simulink model "CrossAR"  (R2020b)
settings: Solver=FixedStepDiscrete  StartTime=0.0  StopTime=99*ModelParam.Samples4Frame  RelTol=1e-3
InitFcn:
  | disp([gcs ': InitFcn']);
  | ModelParam = CrossAR_init([bdroot '/ModelParameters']);
undefined symbols (not defined in the file or in its folder): dfilt
libraries: dspstat3 x17, commchan3 x2, LibCrossAr x2, dspparest3 x2, dspobslib x2, dspsrcs4 x1
Description:
  | % Francesco Conti, Gaetano Scarano, Stefania Colonnese, Mauro Biagi, 2021/01/04%
  | % Copyright: This is published under BSD BSD 3-Clause License
  | 
  | % Copyright (c) 2021, francescoconti748 (Francesco Conti)
  | % All rights reserved, see LICENSE file
  | %
settings Model: Creator=gscarano  LastModifiedBy=conti
settings DataIOCC: LimitDataPoints=on  SaveFormat=Array  SignalLoggingSaveFormat=ModelDataLogs  SaveOutput=off  SignalLogging=off  SaveTime=off  ReturnWorkspaceOutputs=off
settings OptimizationCC: ExpressionDepthLimit=2147483647  LifeSpan=inf
settings DebuggingCC: AlgebraicLoopMsg=error  UnderspecifiedInitializationDetection=Classic  MergeDetectMultiDrivingBlocksExec=none  SolverPrmCheckMsg=warning  SingleTaskRateTransMsg=error  FcnCallInpInsideContextMsg=warning  StateNameClashWarn=warning  SFUnexpectedBacktrackingDiag=warning  SFNoUnconditionalDefaultTransitionDiag=warning  SFExecutionAtInitializationDiag=none  ArithmeticOperatorsInVariantConditions=warning
settings HardwareCC: ProdBitPerPointer=32  ProdBitPerSizeT=32  ProdBitPerPtrDiffT=32  ProdLargestAtomicFloat=None  ProdIntDivRoundTo=Undefined  ProdEndianess=Unspecified  ProdWordSize=32  ProdHWDeviceType=32-bit Generic
settings ModelReferenceCC: PropagateSignalLabelsOutOfModel=off
settings SFSimCC: SimUseLocalCustomCode=off  SimParseCustomCode=off  CustomCodeUndefinedFunction=UseInterfaceOnly
settings RTWCC: RTWUseLocalCustomCode=off
settings CodeAppCC: StateflowObjectComments=on
settings GRTTargetCC: TargetLangStandard=C89/C90 (ANSI)  CombineOutputUpdateFcns=off  GRTInterface=on
settings ConfigComp: CovMetricSettings=dw  CovSaveCumulativeToWorkspaceVar=on  CovSaveSingleToWorkspaceVar=on  CovExternalEMLEnable=off  DVMaxProcessTime=600  DVAutomaticStubbing=off  DVModelCoverageObjectives=MCDC  DVMaxTestCaseSteps=500  DVTestSuiteOptimization=CombinedObjectives  DVDetectActiveLogic=on  DVSaveHarnessModel=on  DVSaveReport=on

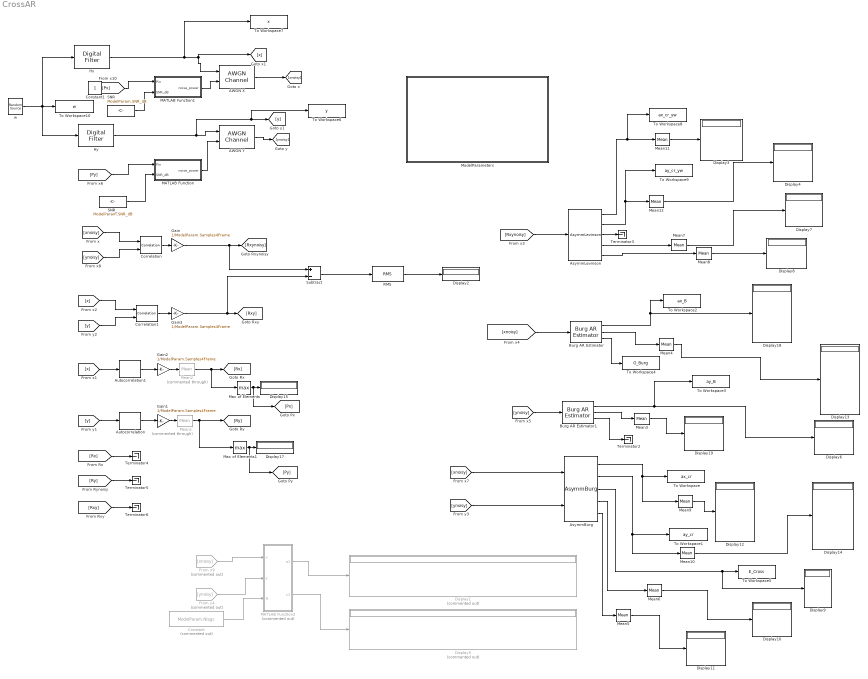
== system CrossAR ==
  AWGN X : commchan3/AWGN Channel  InputProcessing=Columns as channels (frame based)  seed=135  noiseMode=Variance from port  EbNodB=10  EsNodB=10  SNRdB=10  bitsPerSym=1  Ps=1  Tsym=1  variance=ModelParam.NoisePowX
  AWGN Y : commchan3/AWGN Channel  InputProcessing=Columns as channels (frame based)  seed=531  noiseMode=Variance from port  EbNodB=10  EsNodB=10  SNRdB=10  bitsPerSym=1  Ps=1  Tsym=1  variance=ModelParam.NoisePowY
  AsymmBurg : LibCrossAr/AsymmBurg  N=ModelParam.Nlags  Samples4Frame=ModelParam.Samples4Frame
  AsymmLevinson : LibCrossAr/AsymmLevinson  Nlags=ModelParam.Nlags  Samples4Frame=ModelParam.Samples4Frame
  Autocorrelation : dspstat3/Autocorrelation  AllPositiveLags=on  maxlag=1  bias=None  domain=Time  roundingMode=Floor  overflowMode=off  outputDataTypeStr=Inherit: Same as accumulator  outputMin=[]  outputMax=[]  outputLastDataTypeStr=Inherit: Same as accumulator
      settings: SourceProductBaseCode=DS
  Autocorrelation1 : dspstat3/Autocorrelation  AllPositiveLags=on  maxlag=1  bias=None  domain=Time  roundingMode=Floor  overflowMode=off  outputDataTypeStr=Inherit: Same as accumulator  outputMin=[]  outputMax=[]  outputLastDataTypeStr=Inherit: Same as accumulator
      settings: SourceProductBaseCode=DS
  Burg AR Estimator : dspparest3/Burg AR Estimator  fcn=A and K  inheritOrder=off  ord=ModelParam.Nlags
      settings: SourceProductBaseCode=DS
  Burg AR Estimator1 : dspparest3/Burg AR Estimator  fcn=A and K  inheritOrder=off  ord=ModelParam.Nlags
      settings: SourceProductBaseCode=DS
  Constant : Constant  Commented=on  Value=ModelParam.Nlags
  Correlation : dspstat3/Correlation  domain=Fastest  roundingMode=Floor  overflowMode=off  outputDataTypeStr=Inherit: Same as accumulator  outputMin=[]  outputMax=[]  outputLastDataTypeStr=Inherit: Same as accumulator
      settings: SourceProductBaseCode=DS
  Correlation1 : dspstat3/Correlation  domain=Fastest  roundingMode=Floor  overflowMode=off  outputDataTypeStr=Inherit: Same as accumulator  outputMin=[]  outputMax=[]  outputLastDataTypeStr=Inherit: Same as accumulator
      settings: SourceProductBaseCode=DS
  Display1 : Display  Commented=on
  Display{2..4,6..15,17..19} (16 alike) : Display
  Display5 : Display  Commented=on
  From x9 : From  Commented=on  GotoTag=xnoisy
  From y4 : From  Commented=on  GotoTag=ynoisy
  Gain{,1..3} (4 alike) : Gain  Gain=1/ModelParam.Samples4Frame
  Hx : dspobslib/Digital Filter  TypePopup=IIR (all poles)  IIRFiltStruct=Direct form II transposed  AllPoleFiltStruct=Direct form  FIRFiltStruct=Direct form  CoeffSource=Specify via dialog  NumCoeffs=[1 2]  DenCoeffs=ModelParam.Ax  BiQuadCoeffs=[1 0.3 0.4 1 0.1 0.2]  LatticeCoeffs=[.9 -0.5]  denIgnore=on  FiltPerSampPopup=One filter per frame  IC=0  ICnum=0  ICden=0  roundingMode=Floor  overflowMode=off  ScaleValues=1  scaleValueFracLength=14  stageInFracLength=15  stageOutFracLength=15  FilterSource=Specify via dialog  dfiltObjectName=dfilt.dffir([1 2 1])  InputProcessing=Columns as channels (frame based)
      settings: SourceProductBaseCode=DS
  Hy : dspobslib/Digital Filter  TypePopup=IIR (all poles)  IIRFiltStruct=Direct form II transposed  AllPoleFiltStruct=Direct form  FIRFiltStruct=Direct form  CoeffSource=Specify via dialog  NumCoeffs=[1 2]  DenCoeffs=ModelParam.Ay  BiQuadCoeffs=[1 0.3 0.4 1 0.1 0.2]  LatticeCoeffs=[.8 0.3]  denIgnore=on  FiltPerSampPopup=One filter per frame  IC=0  ICnum=0  ICden=0  roundingMode=Floor  overflowMode=off  ScaleValues=1  scaleValueFracLength=14  stageInFracLength=15  stageOutFracLength=15  FilterSource=Specify via dialog  dfiltObjectName=dfilt.dffir([1 2 1])  InputProcessing=Columns as channels (frame based)
      settings: SourceProductBaseCode=DS
  MATLAB Function : MATLAB Function  TreatAsAtomicUnit=on
  MATLAB Function1 : MATLAB Function  TreatAsAtomicUnit=on
  MATLAB Function2 : MATLAB Function  Commented=on  TreatAsAtomicUnit=on  mask{N=ModelParam.Nlags}
  Max of Elements : MinMax  Function=max
  Max of Elements1 : MinMax  Function=max
  Mean1 : dspstat3/Mean  Commented=through  run=on  reset_popup=None  directionMode=Each column  dimension=1  roiEnable=off  roiType=Rectangles  roiPortion=Entire ROI  roiOutput=Individual statistics for each ROI  roiFlag=off  roundingMode=Floor  overflowMode=off  outputDataTypeStr=Inherit: Same as accumulator  outputMin=[]  outputMax=[]  outputLastDataTypeStr=Inherit: Same as accumulator
  Mean{3..12} (10 alike) : dspstat3/Mean  run=on  reset_popup=None  directionMode=Each column  dimension=1  roiEnable=off  roiType=Rectangles  roiPortion=Entire ROI  roiOutput=Individual statistics for each ROI  roiFlag=off  roundingMode=Floor  overflowMode=off  outputDataTypeStr=Inherit: Same as accumulator  outputMin=[]  outputMax=[]  outputLastDataTypeStr=Inherit: Same as accumulator
  Mean2 : dspstat3/Mean  Commented=through  run=on  reset_popup=None  directionMode=Each column  dimension=1  roiEnable=off  roiType=Rectangles  roiPortion=Entire ROI  roiOutput=Individual statistics for each ROI  roiFlag=off  roundingMode=Floor  overflowMode=off  outputDataTypeStr=Inherit: Same as accumulator  outputMin=[]  outputMax=[]  outputLastDataTypeStr=Inherit: Same as accumulator
  ModelParameters : Subsystem  mask(Model Parameters){ExcitationPow=1, Samples4Frame=2048, Nlags=4, SigPow=1, Poles_x=[ 0.7, pi/12; 0.7, -pi/12; 0.7, pi/4; 0.7, -pi/4], Poles_y=[ 0.7, pi/12; 0.7, -pi/12; 0.7, pi/4; 0.7, -pi/4], Ax=[1     -2.3422      2.3187     -1.1477      0.2401], Ay=[1     -2.3422      2.3187     -1.1477      0.2401], SNR_dB=15}
      mask prompts: ExcitationPow "Excitation Power"; SigPow "Signal Power"; Poles_x "Poles_x [vettore]"; Poles_y "Poles_y [vettore]"
      mask help: Model Parameters
      mask Help:
      | % Francesco Conti, Gaetano Scarano, Stefania Colonnese, Mauro Biagi, 2021/01/04%
      | % Copyright: This is published under BSD BSD 3-Clause License
      | 
      | % Copyright (c) 2021, francescoconti748 (Francesco Conti)
      | % All rights reserved, see LICENSE file
      | %
      mask Callback Poles_x:
      | p = eval(get_param(gcb, 'Poles_x'));
      | [b,a] = zp2tf(1, p(:, 1).*exp(j*p(:,2)), 1 ) ;
      | set_param(gcb, 'Ax', ['[' num2str(a) ']' ]);
      mask Callback Poles_y:
      | p = eval(get_param(gcb, 'Poles_y'));
      | [b,a] = zp2tf(1, p(:, 1).*exp(j*p(:,2)), 1 ) ;
      | set_param(gcb, 'Ay', ['[' num2str(a) ']' ]);
      mask DialogControl ParameterTabVar0 Prompt: Excitation Parameters
      mask DialogControl ParameterTabVar01 Prompt: Simulation Parameters
      mask DialogControl ParameterTabVar012 Prompt: Signal Parameters
      mask DialogControl ParameterTabVar0123 Prompt: Noise
      mask Display:
      | text(0.25,.96,'Simulation Parameters');
      | text(0.1,.90,['Samples4Frame:' get_param(gcb,'Samples4Frame')]);
      | text(0.25,.76,'Excitation Parameters');
      | %text(0.1,.70,['Ecitation Power: ' get_param(gcb,'ExcitationPow')]);
      | text(0.1,.70,['SNR(dB): ' get_param(gcb,'SNR_dB')]);
      | text(0.25,.56,'Signal Parameters');
      | text(0.1,.50,['Power: ' get_param(gcb,'SigPow')]);
      | text(0.1,.44,['Nlags: ' get_param(gcb,'Nlags')]);
      | text(0.1,.38,['Poles_x: ' get_param(gcb,'Poles_x')]);
      | text(0.1,.32,['Poles_y: ' get_param(gcb,'Poles_y')]);
      | text(0.1,.26,['Ax: ' get_param(gcb,'Ax')]);
      | text(0.1,.20,['Ay: ' get_param(gcb,'Ay')]);
  RMS : dspstat3/RMS  run=off  directionMode=Each column  dimension=1  InputProcessing=Columns as channels (frame based)  reset_popup=None
  SNR : Constant  Value=ModelParam.SNR_dB
  SNR_ : Constant  Value=ModelParam.SNR_dB
  Subtract : Sum  Inputs=+-
  Terminator{2..6} (5 alike) : Terminator
  To Workspace : ToWorkspace  VariableName=ax_cr  SaveFormat=Timeseries  SampleTime=-1
  To Workspace1 : ToWorkspace  VariableName=ay_cr  SaveFormat=Timeseries  SampleTime=-1
  To Workspace10 : ToWorkspace  VariableName=w  SaveFormat=Timeseries  SampleTime=-1
  To Workspace2 : ToWorkspace  VariableName=ax_B  SaveFormat=Timeseries  SampleTime=-1
  To Workspace3 : ToWorkspace  VariableName=ay_B  SaveFormat=Timeseries  SampleTime=-1
  To Workspace4 : ToWorkspace  VariableName=G_Burg  SaveFormat=Timeseries  SampleTime=-1
  To Workspace5 : ToWorkspace  VariableName=E_Cross  SaveFormat=Timeseries  SampleTime=-1
  To Workspace6 : ToWorkspace  VariableName=y  SaveFormat=Timeseries  SampleTime=-1
  To Workspace7 : ToWorkspace  VariableName=x  SaveFormat=Timeseries  SampleTime=-1
  To Workspace8 : ToWorkspace  VariableName=ax_cr_yw  SaveFormat=Timeseries  SampleTime=-1
  To Workspace9 : ToWorkspace  VariableName=ay_cr_yw  SaveFormat=Timeseries  SampleTime=-1
  w : dspsrcs4/Random Source  SrcType=Gaussian  NormMethod=Ziggurat  CltLength=12  MinVal=0  MaxVal=1  MeanVal=0  VarVal=ModelParam.ExcitationPow  RepMode=Specify seed  rawSeed=3  IsInherit=off  SampMode=Discrete  SampTime=1  SampFrame=ModelParam.Samples4Frame  DataType=Double  OutComplex=Real  OutputFrames=on
  Constant1 : Constant  IOType=siggen
  wires:
  Hx/1 -> To Workspace7/1, AWGN X/1, [x]
  Hy/1 -> AWGN Y/1, To Workspace6/1, [y]
  AWGN X/1 -> [xnoisy]
  AWGN Y/1 -> [ynoisy]
  [xnoisy] -> Correlation/1
  [ynoisy] -> Correlation/2
  Correlation/1 -> Gain/1
  Autocorrelation/1 -> Gain1/1
  Gain/1 -> [Rxynoisy], Subtract/1
  Autocorrelation1/1 -> Gain2/1
  [y] -> Autocorrelation/1
  [x] -> Autocorrelation1/1
  [x] -> Correlation1/1
  [y] -> Correlation1/2
  Correlation1/1 -> Gain3/1
  Gain3/1 -> [Rxy], Subtract/2
  Subtract/1 -> RMS/1
  RMS/1 -> Display2/1
  [Rxynoisy] -> AsymmLevinson/1
  AsymmLevinson/1 -> To Workspace8/1, Mean11/1
  AsymmLevinson/2 -> To Workspace9/1, Mean12/1
  [xnoisy] -> Burg AR Estimator/1
  Burg AR Estimator1/1 -> To Workspace3/1, Display6/1
  [ynoisy] -> Burg AR Estimator1/1
  AsymmLevinson/4 -> Mean7/1
  AsymmLevinson/5 -> Mean8/1
  Mean6/1 -> Display10/1
  Mean5/1 -> Display11/1
  w/1 -> To Workspace10/1, Hy/1, Hx/1
  [ynoisy] -> AsymmBurg/2
  Burg AR Estimator1/3 -> Terminator2/1
  AsymmLevinson/3 -> Terminator3/1
  [Rx] -> Terminator4/1
  [Ry] -> Terminator5/1
  [Rxy] -> Terminator6/1
  Mean4/1 -> Display13/1
  [xnoisy] -> AsymmBurg/1
  AsymmBurg/3 -> Display9/1, To Workspace5/1
  AsymmBurg/4 -> Mean6/1
  AsymmBurg/2 -> Mean10/1, To Workspace1/1
  AsymmBurg/1 -> To Workspace/1, Mean9/1
  Max of Elements/1 -> [Px], Display15/1
  Gain1/1 -> Mean1/1
  Gain2/1 -> Mean2/1
  Mean2/1 -> Max of Elements/1, [Rx]
  Max of Elements1/1 -> [Py], Display17/1
  Mean1/1 -> Max of Elements1/1, [Ry]
  Burg AR Estimator/2 -> Mean4/1
  Burg AR Estimator/1 -> To Workspace2/1, Display18/1
  Burg AR Estimator1/2 -> Mean3/1
  Mean3/1 -> Display19/1
  Mean7/1 -> Display7/1
  Mean8/1 -> Display8/1
  Burg AR Estimator/3 -> To Workspace4/1
  Mean9/1 -> Display12/1
  Mean10/1 -> Display14/1
  Mean11/1 -> Display3/1
  Mean12/1 -> Display4/1
  AsymmBurg/5 -> Mean5/1
  [Py] -> MATLAB Function/1(Pin)
  SNR_/1 -> MATLAB Function/2(SNR_dB)
  MATLAB Function/1(noise_power) -> AWGN Y/2
  [Px] -> MATLAB Function1/1(Pin)
  MATLAB Function1/1(noise_power) -> AWGN X/2
  SNR/1 -> MATLAB Function1/2(SNR_dB)
  From y4/1 -> MATLAB Function2/2(y)
  From x9/1 -> MATLAB Function2/1(x)
  MATLAB Function2/1(a1) -> Display1/1
  Constant/1 -> MATLAB Function2/3(N)
  MATLAB Function2/2(c1) -> Display5/1

== system CrossAR/ModelParameters ==

== matlab function CrossAR/MATLAB Function1 ==
  data: Pin input; noise_power output; SNR_dB input
function noise_power = fcn(Pin, SNR_dB)

    u = Pin*10^(-SNR_dB/10);

noise_power = u;

== matlab function CrossAR/MATLAB Function ==
  data: Pin input; noise_power output; SNR_dB input
function noise_power = fcn(Pin, SNR_dB)

    u = Pin*10^(-SNR_dB/10);

noise_power = u;

== matlab function CrossAR/MATLAB Function2 ==
  data: x input; a1 output size=100 [0..100]; y input; N input; c1 output size=100
function [a1, c1] = fcn(x, y, N)
    a = zeros( 2, 100);
    a1 = zeros(100, 1);
    c1 = zeros(100,1);
    coder.varsize("a", [2, 100])
    
    multi_input = [x, y];

    a = mvar( multi_input, N);
    a1(1:N+1) = [1, -a( 1, 1:2:2*(N) )];
    c1(1:N+1) = [1, -a( 2, 1 + 1:2:2*(N) )];
